simulink model "simulate_OFDM_FFT_transceiver"  (R2017a)
settings: Solver=VariableStepAuto  StartTime=0.0  StopTime=1  RelTol=1e-3
InitFcn:
  | Ts = 1/1000; % symbol time in serial data stream
  | N = 8;  % length of FFT/IFFT
  | T = N*Ts; % symbol time in parallel (OFDM) data stream
libraries: commdigbbndpm3 x2, dspxfrm3 x2, dspindex x2, commchan3 x1, commrandsrc3 x1, simulink x1
settings Model: Creator=prust  LastModifiedBy=prust

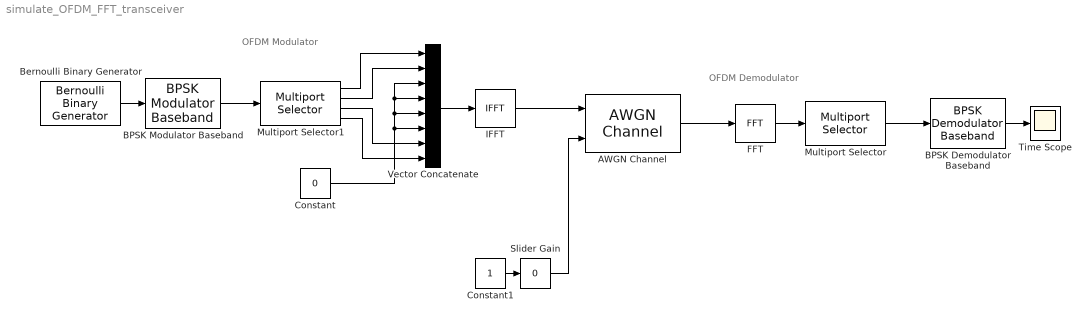
== system simulate_OFDM_FFT_transceiver ==
  note: OFDM Demodulator
  note: OFDM Modulator
  AWGN Channel : commchan3/AWGN Channel  InputProcessing=Columns as channels (frame based)  seed=67  noiseMode=Variance from port  EbNodB=10  EsNodB=10  SNRdB=10  bitsPerSym=1  Ps=1  Tsym=1  variance=1
  BPSK Demodulator Baseband : commdigbbndpm3/BPSK Demodulator Baseband  DecType=Hard decision  VarSource=Dialog  Variance=1  Ph=0  outDtype=Inherit via internal rule  derotateFactorWordLen=16  derotateFactorDataTypeStr=Inherit: Same word length as input  derotateFactorLastDataTypeStr=Inherit: Same word length as input
  BPSK Modulator Baseband : commdigbbndpm3/BPSK Modulator Baseband  Ph=0  outDtype=double  outWordLen=16  outUDDataType=sfix(16)  outFracLenMode=Best precision  outFracLen=15  outDataTypeStr=double  outLastDataTypeStr=double
  Bernoulli Binary Generator : commrandsrc3/Bernoulli Binary Generator  ProbabilityOfZero=0.5  SeedSource=Auto  Seed=0  SampleTime=1/1000  SamplesPerFrame=4  OutputDataType=double  SimulateUsing=Interpreted execution
  Constant : Constant  Value=0
  Constant1 : Constant
  FFT : dspxfrm3/FFT  FFTImplementation=Auto  CompMethod=Table lookup  TableOpt=NEW  TableOptActive=Speed  BitRevOrder=off  Normalize=off  InheritFFTLength=on  FFTLength=64  WrapInput=on  roundingMode=Floor  overflowMode=off  firstCoeffDataTypeStr=Inherit: Same word length as input  firstCoeffLastDataTypeStr=Inherit: Same word length as input  outputMin=[]  outputMax=[]
  IFFT : dspxfrm3/IFFT  FFTImplementation=Auto  CompMethod=Table lookup  TableOpt=NEW  TableOptActive=Speed  BitRevOrder=off  cs_in=off  Normalize=on  InheritFFTLength=on  FFTLength=64  WrapInput=on  mode=Complex  outSamplingMode=Sample based  roundingMode=Floor  overflowMode=off  firstCoeffDataTypeStr=Inherit: Same word length as input  firstCoeffLastDataTypeStr=Inherit: Same word length as input  outputMin=[]  outputMax=[]
      settings: SourceProductName=DSP System Toolbox
  Multiport Selector : dspindex/Multiport Selector  rowsOrCols=Rows  idxCellArray={ [1 2 7 8] }  idxErrMode=Clip Index
  Multiport Selector1 : dspindex/Multiport Selector  rowsOrCols=Rows  idxCellArray={ 1,2,3,4 }  idxErrMode=Clip Index
  Slider Gain : simulink/Math Operations/Slider Gain  gain=0  low=0  high=1
  Time Scope : Scope
  Vector Concatenate : Concatenate  NumInputs=8
  wires:
  Bernoulli Binary Generator/1 -> BPSK Modulator Baseband/1
  Vector Concatenate/1 -> IFFT/1
  IFFT/1 -> AWGN Channel/1
  Constant1/1 -> Slider Gain/1
  Slider Gain/1 -> AWGN Channel/2
  AWGN Channel/1 -> FFT/1
  FFT/1 -> Multiport Selector/1
  Multiport Selector/1 -> BPSK Demodulator Baseband/1
  BPSK Demodulator Baseband/1 -> Time Scope/1
  BPSK Modulator Baseband/1 -> Multiport Selector1/1
  Multiport Selector1/1 -> Vector Concatenate/1
  Multiport Selector1/2 -> Vector Concatenate/2
  Multiport Selector1/4 -> Vector Concatenate/8
  Multiport Selector1/3 -> Vector Concatenate/7
  Constant/1 -> Vector Concatenate/6, Vector Concatenate/3, Vector Concatenate/4, Vector Concatenate/5
